simulink model "obj_atteint_r2019b"  (R2019b)
settings: Solver=FixedStepAuto  StartTime=0.0  StopTime=20000  FixedStep=1  RelTol=1e-3
values from neighbouring files (symbols this model uses):
  A = [0 0 1 0 ... (first row only)    [Params.m]    (also in tests.m)
  B = [0 0;0 0;1 0;0 1]    [Params.m]    (also in tests.m)
  C = [1 0 0 0;0 1 0 0]    [Params.m]    (also in tests.m)
  D = zeros(2)    [Params.m]    (also in tests.m)
  hold_points = [ ... (first row only)    [Params.m]    (also in tests.m)
  Kc = lqr(A,B,Q,R)    [Params.m]    (also in closing.m; tests.m)
  Kf = Kf'    [Params.m]    (also in closing.m; tests.m)
settings Model: Creator=Kevin  LastModifiedBy=aug19

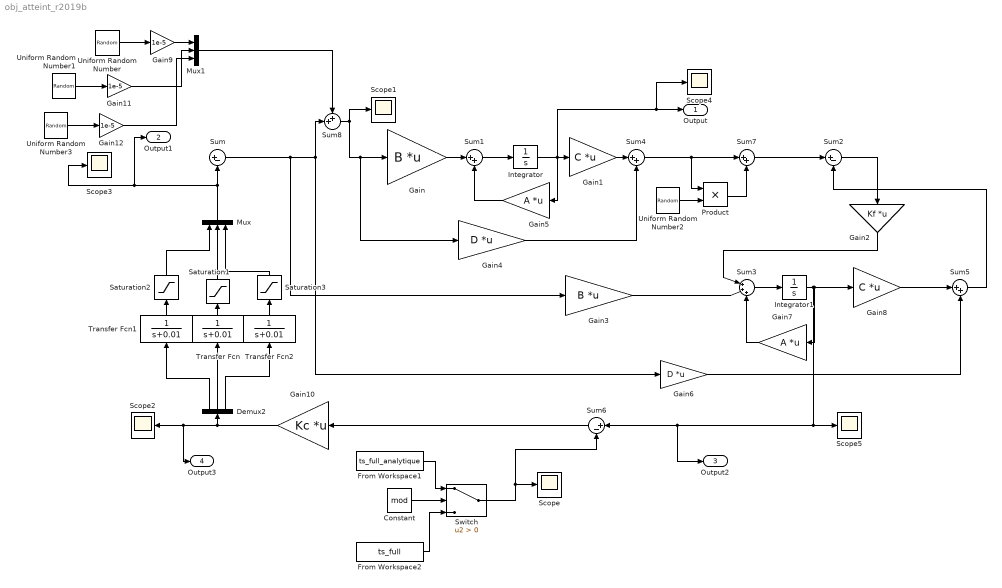
== system obj_atteint_r2019b ==
  Constant : Constant  Value=mod
  Demux2 : Demux  Outputs=3
  From Workspace1 : FromWorkspace  VariableName=ts_full_analytique  SampleTime=-1  OutputAfterFinalValue=Holding final value
  From Workspace2 : FromWorkspace  VariableName=ts_full  SampleTime=-1  OutputAfterFinalValue=Holding final value
  Gain : Gain  Gain=B  Multiplication=Matrix(K*u) (u vector)
  Gain1 : Gain  Gain=C  Multiplication=Matrix(K*u) (u vector)
  Gain10 : Gain  Gain=Kc  Multiplication=Matrix(K*u) (u vector)
  Gain11 : Gain  Gain=1e-5
  Gain12 : Gain  Gain=1e-5
  Gain2 : Gain  Gain=Kf  Multiplication=Matrix(K*u) (u vector)
  Gain3 : Gain  Gain=B  Multiplication=Matrix(K*u) (u vector)
  Gain4 : Gain  Gain=D  Multiplication=Matrix(K*u) (u vector)
  Gain5 : Gain  Gain=A  Multiplication=Matrix(K*u) (u vector)
  Gain6 : Gain  Gain=D  Multiplication=Matrix(K*u) (u vector)
  Gain7 : Gain  Gain=A  Multiplication=Matrix(K*u) (u vector)
  Gain8 : Gain  Gain=C  Multiplication=Matrix(K*u) (u vector)
  Gain9 : Gain  Gain=1e-5
  Integrator : Integrator  InitialCondition=hold_points(1,:)
  Integrator1 : Integrator  InitialCondition=hold_points(1,:)
  Mux : Mux  Inputs=3
  Mux1 : Mux  Inputs=3
  Product : Product
  Saturation1 : Saturate  UpperLimit=0.01  LowerLimit=-0.01
  Saturation2 : Saturate  UpperLimit=0.01  LowerLimit=-0.01
  Saturation3 : Saturate  UpperLimit=0.01  LowerLimit=-0.01
  Scope{,1..5} (6 alike) : Scope
  Sum : Sum  Inputs=|+-
  Sum{1,4..5,7} (4 alike) : Sum  Inputs=|++
  Sum2 : Sum  Inputs=|+-
  Sum3 : Sum  Inputs=|+++
  Sum6 : Sum  Inputs=|+-
  Sum8 : Sum  Inputs=++|
  Switch : Switch  Criteria=u2 > Threshold
  Transfer Fcn : TransferFcn  Numerator=1  Denominator=[1 0.01]
  Transfer Fcn1 : TransferFcn  Numerator=1  Denominator=[1 0.01]
  Transfer Fcn2 : TransferFcn  Numerator=1  Denominator=[1 0.01]
  Uniform Random Number : UniformRandomNumber  SampleTime=1
  Uniform Random Number1 : UniformRandomNumber  SampleTime=1
  Uniform Random Number2 : UniformRandomNumber  Minimum=-0.1  Maximum=0.1  SampleTime=1
  Uniform Random Number3 : UniformRandomNumber  SampleTime=1
  Output : Outport  SignalName=etat
  Output1 : Outport  Port=2  SignalName=commande
  Output2 : Outport  Port=3  SignalName=etat_est
  Output3 : Outport  Port=4  SignalName=commande
  wires:
  Sum/1 -> Sum8/2, Gain6/1, Gain3/1
  Sum1/1 -> Integrator/1
  Gain/1 -> Sum1/1
  Integrator/1 -> Gain5/1, Scope4/1, Output/1, Gain1/1
  Sum2/1 -> Gain2/1
  Gain2/1 -> Sum3/1
  Gain3/1 -> Sum3/2
  Gain1/1 -> Sum4/1
  Sum7/1 -> Sum2/1
  Gain4/1 -> Sum4/2
  Gain5/1 -> Sum1/2
  Sum3/1 -> Integrator1/1
  Integrator1/1 -> Gain8/1, Gain7/1, Scope5/1, Output2/1, Sum6/1
  Gain8/1 -> Sum5/1
  Gain6/1 -> Sum5/2
  Gain7/1 -> Sum3/3
  Sum5/1 -> Sum2/2
  Sum6/1 -> Gain10/1
  Switch/1 -> Sum6/2, Scope/1
  Uniform Random Number/1 -> Gain9/1
  Gain9/1 -> Mux1/1
  Sum8/1 -> Scope1/1, Gain4/1, Gain/1
  Mux1/1 -> Sum8/1
  Uniform Random Number1/1 -> Gain11/1
  Gain11/1 -> Mux1/2
  Product/1 -> Sum7/2
  Sum4/1 -> Product/1, Sum7/1
  Uniform Random Number2/1 -> Product/2
  Gain10/1 -> Demux2/1, Output3/1, Scope2/1
  Demux2/1 -> Transfer Fcn1/1
  Demux2/2 -> Transfer Fcn/1
  From Workspace2/1 -> Switch/3
  From Workspace1/1 -> Switch/1
  Constant/1 -> Switch/2
  Demux2/3 -> Transfer Fcn2/1
  Gain12/1 -> Mux1/3
  Uniform Random Number3/1 -> Gain12/1
  Mux/1 -> Scope3/1, Output1/1, Sum/2
  Transfer Fcn1/1 -> Saturation2/1
  Saturation2/1 -> Mux/1
  Transfer Fcn/1 -> Saturation1/1
  Transfer Fcn2/1 -> Saturation3/1
  Saturation3/1 -> Mux/3
  Saturation1/1 -> Mux/2
